simulink model "chap7_4sim"  (R2019a)
settings: Solver=VariableStepAuto  StartTime=0.0  StopTime=10.0  RelTol=1e-3
settings Model: Creator=zkibria  LastModifiedBy=zkibria

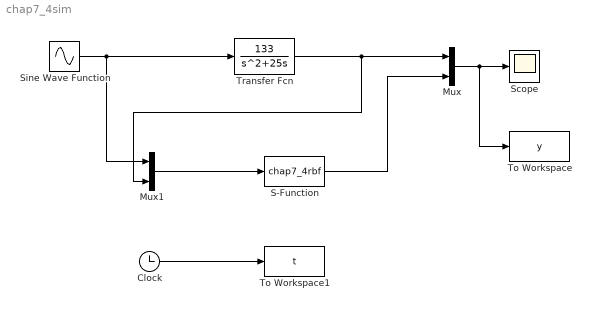
== system chap7_4sim ==
  Clock : Clock
  Mux : Mux  Inputs=2
  Mux1 : Mux  Inputs=2
  S-Function : S-Function  FunctionName=chap7_4rbf  SFunctionDeploymentMode=off  EnableBusSupport=off
  Scope : Scope
  Sine Wave Function : Sin  SampleTime=0
  To Workspace : ToWorkspace  VariableName=y  SaveFormat=Timeseries  SampleTime=-1
  To Workspace1 : ToWorkspace  VariableName=t  SaveFormat=Timeseries  SampleTime=-1
  Transfer Fcn : TransferFcn  Numerator=[133]  Denominator=[1 25 0]
  wires:
  Sine Wave Function/1 -> Transfer Fcn/1, Mux1/1
  Transfer Fcn/1 -> Mux1/2, Mux/1
  Mux/1 -> To Workspace/1, Scope/1
  Mux1/1 -> S-Function/1
  S-Function/1 -> Mux/2
  Clock/1 -> To Workspace1/1
